simulink model "generalized_plant_M"  (R2013a)
settings: Solver=ode45  StartTime=0.0  StopTime=10.0  RelTol=1e-3
values from neighbouring files (symbols this model uses):
  Ga = 3    [a2_data_input_examsim1.m]    (also in a2_data_input_examsim2.m = 1; a2_data_input_hw3.m = 0.095; a2_data_input_mdcs_h5_v1_stud_p1.m = 0.095; a2_data_input_mdcs_h5_v1_stud_p4.m = 0.006)
  Gf = Gr/(Kd*Gs)    [a3_process_input.m]
  Gr = 1    [a2_data_input_examsim1.m]    (also in a2_data_input_examsim2.m; a2_data_input_hw3.m; a2_data_input_mdcs_h5_v1_stud_p1.m; a2_data_input_mdcs_h5_v1_stud_p4.m)
  Gs = 1    [a2_data_input_examsim1.m]    (also in a2_data_input_examsim2.m = 5; a2_data_input_hw3.m; a2_data_input_mdcs_h5_v1_stud_p1.m; a2_data_input_mdcs_h5_v1_stud_p4.m)
  Kd = 2    [a2_data_input_examsim1.m]    (also in a2_data_input_examsim2.m = 1; a2_data_input_hw3.m = 1; a2_data_input_mdcs_h5_v1_stud_p1.m = 1; a2_data_input_mdcs_h5_v1_stud_p4.m = 1)
undefined symbols (not defined in the file or in its folder): Gp, W1, W2
settings Model: Creator=Mauricio  LastModifiedBy=s171105
settings OptimizationCC: ExpressionDepthLimit=2147483647
settings DebuggingCC: StrictBusMsg=Warning
settings GRTTargetCC: CombineOutputUpdateFcns=off  GRTInterface=on

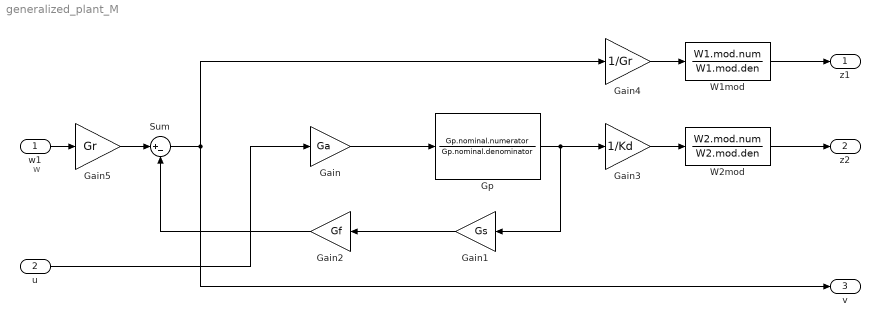
== system generalized_plant_M ==
  note: w
  w1 : Inport
  u : Inport  Port=2
  Gain : Gain  Gain=Ga
  Gain1 : Gain  Gain=Gs
  Gain2 : Gain  Gain=Gf
  Gain3 : Gain  Gain=1/Kd
  Gain4 : Gain  Gain=1/Gr
  Gain5 : Gain  Gain=Gr
  Gp : TransferFcn  Numerator=Gp.nominal.numerator  Denominator=Gp.nominal.denominator
  Sum : Sum  Inputs=|+-
  W1mod : TransferFcn  Numerator=W1.mod.num  Denominator=W1.mod.den
  W2mod : TransferFcn  Numerator=W2.mod.num  Denominator=W2.mod.den
  z1 : Outport
  z2 : Outport  Port=2
  v : Outport  Port=3
  wires:
  Gp/1 -> Gain1/1, Gain3/1
  W1mod/1 -> z1/1
  W2mod/1 -> z2/1
  u/1 -> Gain/1
  w1/1 -> Gain5/1
  Sum/1 -> v/1, Gain4/1
  Gain/1 -> Gp/1
  Gain2/1 -> Sum/2
  Gain1/1 -> Gain2/1
  Gain3/1 -> W2mod/1
  Gain4/1 -> W1mod/1
  Gain5/1 -> Sum/1
